simulink model "prelab"  (R2025b)
settings: Solver=ode45  StartTime=0.0  StopTime=3  MaxStep=0.001  RelTol=1e-3
settings Model: Creator=eonuf  LastModifiedBy=eonuf

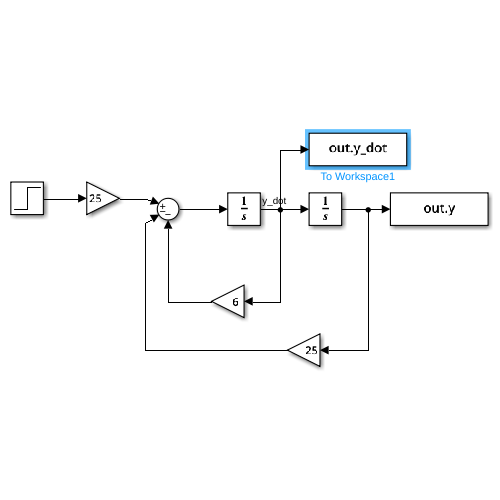
[thumbnail: Simulink's stored preview of the top-level diagram]
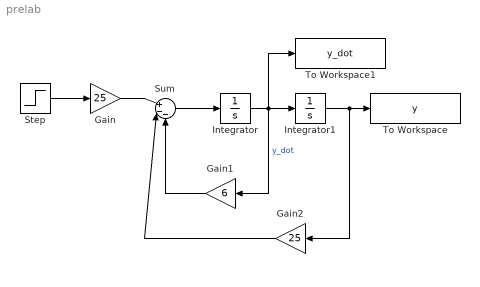
== system prelab ==
  Gain : Gain  Gain=25
  Gain1 : Gain  Gain=6
  Gain2 : Gain  Gain=25
  Integrator : Integrator
  Integrator1 : Integrator
  Step : Step  Time=0  SampleTime=0
  Sum : Sum  Inputs=|+--
  To Workspace : ToWorkspace  VariableName=y  SampleTime=-1
  To Workspace1 : ToWorkspace  VariableName=y_dot  SampleTime=-1
  wires:
  Gain/1 -> Sum/1
  Integrator/1 -> Gain1/1, To Workspace1/1, Integrator1/1  "y_dot"
  Sum/1 -> Integrator/1
  Integrator1/1 -> To Workspace/1, Gain2/1
  Gain1/1 -> Sum/3
  Gain2/1 -> Sum/2
  Step/1 -> Gain/1
